simulink model "ssupLeg"  (R2014b)
settings: Solver=ode3  StartTime=0.0  StopTime=1  FixedStep=.01  RelTol=1e-3
values from neighbouring files (symbols this model uses):
  alpha = 75    [BslipOriginal.m]
  k = 280    [BslipOriginal.m]
  xf = 0    [BslipOriginal.m]
  xinS = xd1.signals.values(end)    [BslipOriginal.m]
  xp = xd.signals.values(end)-(cos(alpha/180*pi)-xpp)    [BslipOriginal.m]
  yinS = yd1.signals.values(end)    [BslipOriginal.m]
  yp = yd.signals.values(end)    [BslipOriginal.m]
libraries: simulink x1
settings Model: Creator=hamidreza  LastModifiedBy=hamidreza

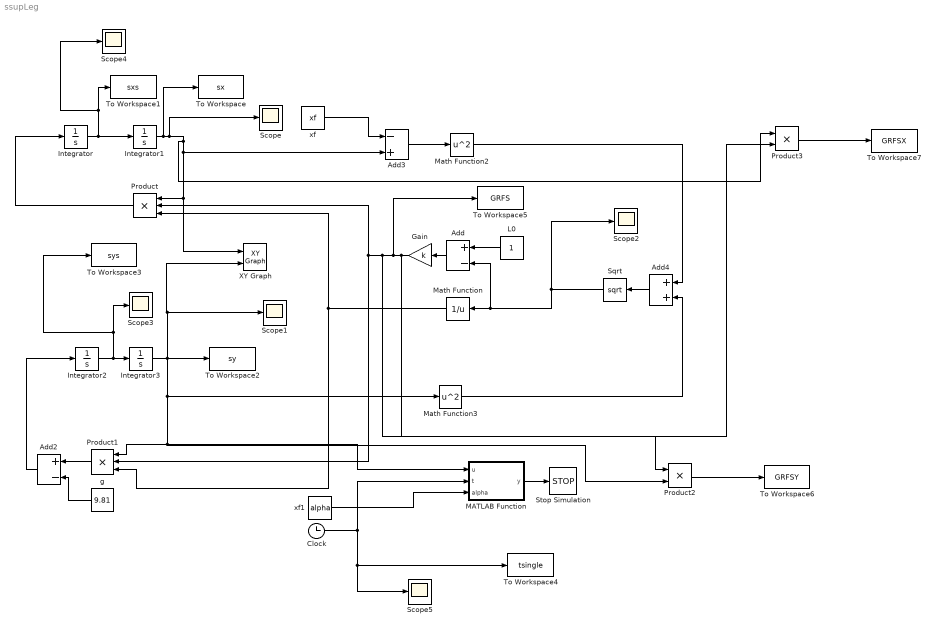
== system ssupLeg ==
  Add : Sum  Inputs=+-
  Add2 : Sum  Inputs=+-
  Add3 : Sum  Inputs=-+
  Add4 : Sum
  Clock : Clock
  Gain : Gain  Gain=k
  Integrator : Integrator  InitialCondition=xinS
  Integrator1 : Integrator  InitialCondition=xp
  Integrator2 : Integrator  InitialCondition=yinS
  Integrator3 : Integrator  InitialCondition=yp
  L0 : Constant
  MATLAB Function : MATLAB Function  TreatAsAtomicUnit=on
  Math Function : Math  Operator=reciprocal  SaturateOnIntegerOverflow=on
  Math Function2 : Math  Operator=square  SaturateOnIntegerOverflow=on
  Math Function3 : Math  Operator=square  SaturateOnIntegerOverflow=on
  Product : Product  Inputs=3
  Product1 : Product  Inputs=3
  Product2 : Product
  Product3 : Product
  Scope{,1..5} (6 alike) : Scope
      Scope settings: TimeRange=0.17  YMin=-0.102  YMax=-0.088
      Scope1 settings: TimeRange=0.11  YMin=0.965  YMax=0.98
      Scope2 settings: TimeRange=0.14  YMin=0.97  YMax=1.005  SaveName=ScopeData2
      Scope3 settings: SaveName=ScopeData3
      Scope4 settings: SaveName=ScopeData4
      Scope5 settings: TimeRange=0.14  YMin=0.97  YMax=1.005  SaveName=ScopeData5
  Sqrt : Sqrt  SaturateOnIntegerOverflow=on
  Stop Simulation : Stop
  To Workspace : ToWorkspace  VariableName=sx  SaveFormat=Structure With Time  SampleTime=-1
  To Workspace1 : ToWorkspace  VariableName=sxs  SaveFormat=Structure With Time  SampleTime=-1
  To Workspace2 : ToWorkspace  VariableName=sy  SaveFormat=Structure With Time  SampleTime=-1
  To Workspace3 : ToWorkspace  VariableName=sys  SaveFormat=Structure With Time  SampleTime=-1
  To Workspace4 : ToWorkspace  VariableName=tsingle  SampleTime=-1
      settings: Save2DSignal=2-D array (concatenate along first dimension)
  To Workspace5 : ToWorkspace  VariableName=GRFS  SaveFormat=Structure With Time  SampleTime=-1
      settings: Save2DSignal=2-D array (concatenate along first dimension)
  To Workspace6 : ToWorkspace  VariableName=GRFSY  SaveFormat=Structure With Time  SampleTime=-1
      settings: Save2DSignal=2-D array (concatenate along first dimension)
  To Workspace7 : ToWorkspace  VariableName=GRFSX  SaveFormat=Structure With Time  SampleTime=-1
      settings: Save2DSignal=2-D array (concatenate along first dimension)
  XY Graph : simulink/Sinks/XY Graph  xmin=-1  xmax=2  ymin=0  ymax=1  st=-1
  g : Constant  Value=9.81
  xf : Constant  Value=xf
  xf1 : Constant  Value=alpha
  wires:
  Integrator/1 -> To Workspace1/1, Scope4/1, Integrator1/1
  Product/1 -> Integrator/1
  Add/1 -> Gain/1
  Integrator2/1 -> Scope3/1, To Workspace3/1, Integrator3/1
  Product1/1 -> Add2/1
  g/1 -> Add2/2
  Add2/1 -> Integrator2/1
  xf/1 -> Add3/1
  Add3/1 -> Math Function2/1
  Math Function2/1 -> Add4/1
  Add4/1 -> Sqrt/1
  Sqrt/1 -> Add/2, Math Function/1, Scope2/1
  L0/1 -> Add/1
  Integrator3/1 -> XY Graph/2, Scope1/1, Product2/2, Product1/1, MATLAB Function/1(u), Math Function3/1, To Workspace2/1
  Clock/1 -> To Workspace4/1, Scope5/1, MATLAB Function/2(t)
  MATLAB Function/1(y) -> Stop Simulation/1
  Math Function3/1 -> Add4/2
  Gain/1 -> Product2/1, To Workspace5/1, Product3/2, Product1/2, Product/2
  Math Function/1 -> Product/3, Product1/3
  Product2/1 -> To Workspace6/1
  Product3/1 -> To Workspace7/1
  Integrator1/1 -> To Workspace/1, Scope/1, Product3/1, Add3/2, Product/1, XY Graph/1
  xf1/1 -> MATLAB Function/3(alpha)

== matlab function ssupLeg/MATLAB Function ==
  data: u input; y output; t input; alpha input
function y = fcn(u,t,alpha)
%#codegen

if and(u-sin(alpha/180*pi)<.001,t>.04)
    y=1;
else
    y=0;

end
